simulink model "sgMdl_IO624_SyncAsync"  (R2024b)
settings: Solver=FixedStepAuto  StartTime=0.0  StopTime=inf  RelTol=1e-3  EnableMultiTasking=on
undefined symbols (not defined in the file): A, Asynchronous, FIFO, ns, PSI5, Triggered, us
libraries: speedgoatlib_IO624 x7
Description:
  | IO624 - PSI5
settings Model: ModifiedByFormat=Speedgoat  SimulationMode=external  ExtModeEnableFloating=off  ExtModeTrigDuration=100000  Creator=Speedgoat  LastModifiedBy=Speedgoat
settings SolverCC: ConcurrentTasks=on  AlgebraicLoopSolver=TrustRegion  PositivePriorityOrder=on  AutoInsertRateTranBlk=on  InsertRTBMode=Never (minimum delay)
settings DataIOCC: SaveFormat=StructureWithTime
settings OptimizationCC: BlockReduction=off  OptimizeBlockIOStorage=off  BufferReuse=off  GlobalBufferReuse=off  ExpressionFolding=off  LocalBlockOutputs=off  OptimizeDataStoreBuffers=off  BusAssignmentInplaceUpdate=off
settings DebuggingCC: InheritedTsInSrcMsg=none  TasksWithSamePriorityMsg=none  ParameterPrecisionLossMsg=none  UnconnectedInputMsg=warning  UnconnectedOutputMsg=warning  UnconnectedLineMsg=warning
settings HardwareCC: ProdBitPerLong=64  ProdLongLongMode=on  ProdHWDeviceType=Intel->x86-64 (Linux 64)
settings ModelReferenceCC: EnableRefExpFcnMdlSchedulingChecks=on
settings SFSimCC: CustomCodeUndefinedFunction=UseInterfaceOnly
settings RTWCC: Description=Speedgoat Real-Time Target Machine  SystemTargetFile=speedgoat.tlc  TemplateMakefile=slrealtime_default_tmf  PostCodeGenCommand=sg.model.build.makeCfg(bdroot, buildInfo);  Toolchain=Simulink Real-Time Toolchain  BuildConfiguration=Faster Runs  TargetLang=C++  GPUComputeCapability=3.5  DLArmComputeVersion=19.05
settings SimulinkRealTimeTargetCC: SubcomponentCodeInterfacePackaging=Reusable function  InstructionSetFMA=off  LogToMDFFile=off  SLRTFileLogMaxRuns=10
settings ConfigComp: CovBoundaryAbsTol=1.0e-5

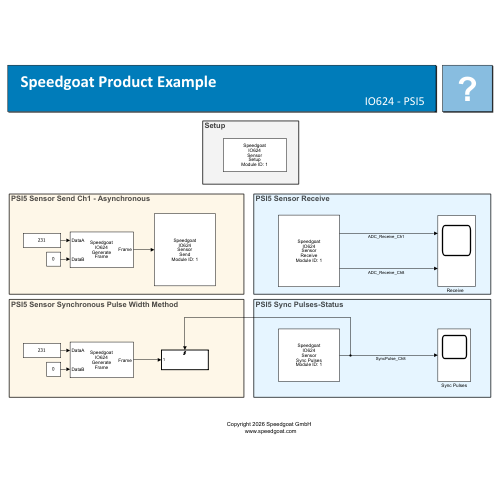
[thumbnail: Simulink's stored preview of the top-level diagram]
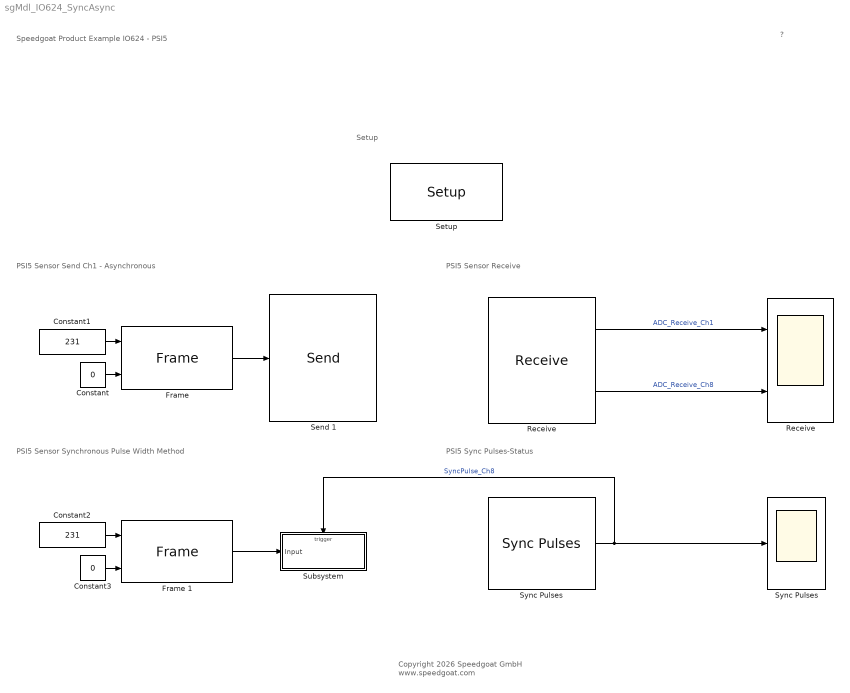
== system sgMdl_IO624_SyncAsync ==
  note: Setup
  note: PSI5 Sensor Send Ch1 - Asynchronous
  note: PSI5 Sensor Receive
  note: PSI5 Sensor Synchronous Pulse Width Method
  note: PSI5 Sync Pulses-Status
  note: Speedgoat Product Example
      | IO624 - PSI5
  note: ?
  note: Copyright 2026 Speedgoat GmbH
      |  www.speedgoat.com
  Constant : Constant  Value=0  OutDataTypeStr=uint16
  Constant1 : Constant  Value=231  OutDataTypeStr=uint32
  Constant2 : Constant  Value=231  OutDataTypeStr=uint32
  Constant3 : Constant  Value=0  OutDataTypeStr=uint16
  "Frame " : speedgoatlib_IO624/Frame   parSizeDataA=7  parSizeDataB=0  parEnableMsging=off  parMsging=[1, 1]  parEnableFrameCtrl=off  parFrameCtrl=[1, 0]  parEnableMsgStatus=off  parMsgStatus=[0, 1]
      settings: SourceProductName=IO624
  Frame 1 : speedgoatlib_IO624/Frame   parSizeDataA=7  parSizeDataB=0  parEnableMsging=off  parMsging=[1, 1]  parEnableFrameCtrl=off  parFrameCtrl=[1, 0]  parEnableMsgStatus=off  parMsgStatus=[0, 1]
      settings: SourceProductName=IO624
  "Receive " : speedgoatlib_IO624/Receive   parModuleId=1  parModuleNumber=624  parSampleTime=5e-5  parPciSlot=-1  parMonitorCh=[1 8]
      settings: SourceProductName=IO624
  "Receive  " : Scope  NumInputPorts=2
  Send 1 : speedgoatlib_IO624/Send   parSendChannels=1  parModuleNumber=624  parModuleId=1  parSampleTime=5e-5  parSendChStatus1=off  parSendChStatus2=off  parSendChStatus3=off  parSendChStatus4=off  parSendChStatus5=off  parSendChStatus6=off  parSendChStatus7=off  parSendChStatus8=off  parSendChannel1=on  parSendChannel2=off  parSendChannel3=off  parSendChannel4=off  parSendChannel5=off  parSendChannel6=off  parSendChannel7=off  parSendChannel8=off  parPciSlot=-1  parCtrChannels=[2 1 1 1 1 1 1 2]  parSendChsStatus=zeros(1,0)  parSendPSI5=[1 1 1 1 2 2 2 2 105 105 105 105 65 65 65 65 1000 500 500 500 500 500 500 1500]
      settings: SourceProductName=IO624
  "Setup " : speedgoatlib_IO624/Setup   parModuleNumber=624  parModuleId=1  parPciSlot=-1  parTriggerSignal=TTL  parChsequence=[1 8]  parCtrChannels=[2 1 1 1 1 1 1 2]  parCtrCh1=PSI5 Sensor Emulator  parMonitorCh1=on  parCtrCh2=Disabled  parMonitorCh2=off  parCtrCh3=Disabled  parMonitorCh3=off  parCtrCh4=Disabled  parMonitorCh4=off  parCtrCh5=Disabled  parMonitorCh5=off  parCtrCh6=Disabled  parMonitorCh6=off  parCtrCh7=Disabled  parMonitorCh7=off  parCtrCh8=PSI5 Sensor Emulator  parMonitorCh8=on  parModuleSetV=[1 2 1 1 1 1 1 1 2]  parCurrentL=[0 14000 10000 0 14000 10000 0 14000 10000 0 14000 10000 10000 14000 17000 10000 14000 17000 10000 14000 17000 10000 14000 17000 0 0 0]  parCh1=[0 0 80 0 0 1000 8600 3000 5 45 2 0 0 0 1 10 1 1]  parCh2=[0 0 0 0 0 0 0 0 0 0 0 0 0 0 0 0 0 0]  parCh3=[0 0 0 0 0 0 0 0 0 0 0 0 0 0 0 0 0 0]  parCh4=[0 0 0 0 0 0 0 0 0 0 0 0 0 0 0 0 0 0]  parCh5=[0 0 0 0 0 0 0 0 0 0 0 0 0 0 0 0 0 0]  parCh6=[0 0 0 0 0 0 0 0 0 0 0 0 0 0 0 0 0 0]  parCh7=[0 0 0 0 0 0 0 0 0 0 0 0 0 0 0 0 0 0]  parCh8=[0 0 80 0 0 1500 8600 3000 5 645 2 0 0 0 1 5 2 1]  parPSI5BusModeCh1=PSI5-A (Asynchronous)  parPSI5NBitsCh1=10  parPSI5SBEnableCh1=Start Bit Enable  parPSI5StartBitSXCh1=[0, 0]  parPSI5DataDTCh1=105  parPSI5PayloadCrcCh1=1  parPSI5UVRCh1=Disable  parPSI5UnderVoltReVTHCh1=3000  psi5ReDetecTimeTTHCh1=5  parPSI5SlotDCh1=45  parPSI5PulseModeCh1=Pulse Width Method  parPSI5FrameLCh1=Frame 2a Long (Nibble)  parPSI5SSVoltageCh1=8600  parAKASpeedPulseCh1=Normal (High Current)  parEnDynSpeedPulseLvlCh1=on  parCustomModeCh1=FIFO-Triggered  parCustomNrFifoFramesCh1=1  parBitRateCh1=125 kbps  parBitTimeBaseCh1=0.1 [us]  parBitTimeFactorCh1=80  textEffBitTimeCh1=8.0 [us]  parPulseTimeBaseCh1="50  [ns]"  parPulseTimeFactorCh1=8  textEffPulseTimeCh1=400.0 [ns]  parCycleTimeDesiredCh1=Choose with Time Base and Time Factor  parCycleTimeBaseCh1="1    [us]"  parCycleTimeFactorCh1=1000  textEffCycleTimeCh1=1000.0 [us]  parEnDynTimingCh1=off  parCLCSettingCh1=Custom  parCLHighCh1=10000  parCLMidCh1=14000  parCLLowCh1=0  parPSI5BusModeCh2=PSI5-A (Asynchronous)  parPSI5NBitsCh2=10  parPSI5SBEnableCh2=Start Bit Enable  parPSI5StartBitSXCh2=[0, 0]  parPSI5DataDTCh2=105  parPSI5PayloadCrcCh2=1  parPSI5UVRCh2=Disable  parPSI5UnderVoltReVTHCh2=3000  psi5ReDetecTimeTTHCh2=5  parPSI5SlotDCh2=0  parPSI5PulseModeCh2=Tooth Gap Method  parPSI5FrameLCh2=Frame 2a Long (Nibble)  parPSI5SSVoltageCh2=0  parAKASpeedPulseCh2=Normal (High Current)  parEnDynSpeedPulseLvlCh2=off  parCustomModeCh2=FIFO-Triggered  parCustomNrFifoFramesCh2=1  parBitRateCh2=125 kbps  parBitTimeBaseCh2=0.1 [us]  parBitTimeFactorCh2=80  textEffBitTimeCh2=8.0 [us]  parPulseTimeBaseCh2="50  [ns]"  parPulseTimeFactorCh2=8  textEffPulseTimeCh2=400.0 [ns]  parCycleTimeDesiredCh2=Choose with Time Base and Time Factor  parCycleTimeBaseCh2="50  [ns]"  parCycleTimeFactorCh2=500  textEffCycleTimeCh2=25000.0 [ns]  parEnDynTimingCh2=off  parCLCSettingCh2=Custom  parCLHighCh2=10000  parCLMidCh2=14000  parCLLowCh2=0  parPSI5BusModeCh3=PSI5-A (Asynchronous)  parPSI5NBitsCh3=10  parPSI5SBEnableCh3=Start Bit Enable  parPSI5StartBitSXCh3=[0, 0]  parPSI5DataDTCh3=105  parPSI5PayloadCrcCh3=487  parPSI5UVRCh3=Disable  parPSI5UnderVoltReVTHCh3=3000  psi5ReDetecTimeTTHCh3=5  parPSI5SlotDCh3=0  parPSI5PulseModeCh3=Tooth Gap Method  parPSI5FrameLCh3=Frame 2a Long (Nibble)  parPSI5SSVoltageCh3=0  parAKASpeedPulseCh3=Normal (High Current)  parEnDynSpeedPulseLvlCh3=off  parCustomModeCh3=FIFO-Triggered  parCustomNrFifoFramesCh3=1  parBitRateCh3=125 kbps  parBitTimeBaseCh3=0.1 [us]  parBitTimeFactorCh3=80  textEffBitTimeCh3=8.0 [us]  parPulseTimeBaseCh3=0.1 [us]  parPulseTimeFactorCh3=8  textEffPulseTimeCh3=0.8 [us]  parCycleTimeDesiredCh3=Choose with Time Base and Time Factor  parCycleTimeBaseCh3="50  [ns]"  parCycleTimeFactorCh3=500  textEffCycleTimeCh3=25000.0 [ns]  parEnDynTimingCh3=off  parCLCSettingCh3=Custom  parCLHighCh3=10000  parCLMidCh3=14000  parCLLowCh3=0  parPSI5BusModeCh4=PSI5-A (Asynchronous)  parPSI5NBitsCh4=10  parPSI5SBEnableCh4=Start Bit Enable  parPSI5StartBitSXCh4=[0, 0]  parPSI5DataDTCh4=105  parPSI5PayloadCrcCh4=487  parPSI5UVRCh4=Disable  parPSI5UnderVoltReVTHCh4=3000  psi5ReDetecTimeTTHCh4=5  parPSI5SlotDCh4=0  parPSI5PulseModeCh4=Tooth Gap Method  parPSI5FrameLCh4=Frame 2a Long (Nibble)  parPSI5SSVoltageCh4=0  parAKASpeedPulseCh4=Normal (High Current)  parEnDynSpeedPulseLvlCh4=off  parCustomModeCh4=FIFO-Triggered  parCustomNrFifoFramesCh4=1  parBitRateCh4=Custom  parBitTimeBaseCh4=0.1 [us]  parBitTimeFactorCh4=80  textEffBitTimeCh4=8.0 [us]  parPulseTimeBaseCh4="50  [ns]"  parPulseTimeFactorCh4=8  textEffPulseTimeCh4=400.0 [ns]  parCycleTimeDesiredCh4=Choose with Time Base and Time Factor  parCycleTimeBaseCh4="50  [ns]"  parCycleTimeFactorCh4=500  textEffCycleTimeCh4=25000.0 [ns]  parEnDynTimingCh4=off  parCLCSettingCh4=Custom  parCLHighCh4=10000  parCLMidCh4=14000  parCLLowCh4=0  parPSI5BusModeCh5=PSI5-U/P (Synchronous without Daisy Chain)  parPSI5NBitsCh5=5  parPSI5SBEnableCh5=Start Bit Enable  parPSI5StartBitSXCh5=[0, 0]  parPSI5DataDTCh5=65  parPSI5PayloadCrcCh5=487  parPSI5UVRCh5=Disable  parPSI5UnderVoltReVTHCh5=3000  psi5ReDetecTimeTTHCh5=5  parPSI5SlotDCh5=0  parPSI5PulseModeCh5=Pulse Width Method  parPSI5FrameLCh5=Frame 2a Long (Nibble)  parPSI5SSVoltageCh5=8600  parAKASpeedPulseCh5=Normal (High Current)  parEnDynSpeedPulseLvlCh5=off  parCustomModeCh5=FIFO-Triggered  parCustomNrFifoFramesCh5=1  parBitRateCh5=125 kbps  parBitTimeBaseCh5=0.1 [us]  parBitTimeFactorCh5=80  textEffBitTimeCh5=8.0 [us]  parPulseTimeBaseCh5="50  [ns]"  parPulseTimeFactorCh5=8  textEffPulseTimeCh5=400.0 [ns]  parCycleTimeDesiredCh5=Choose with Time Base and Time Factor  parCycleTimeBaseCh5="50  [ns]"  parCycleTimeFactorCh5=500  textEffCycleTimeCh5=25000.0 [ns]  parEnDynTimingCh5=off  parCLCSettingCh5=Custom  parCLHighCh5=17000  parCLMidCh5=14000  parCLLowCh5=10000  parPSI5BusModeCh6=PSI5-U/P (Synchronous without Daisy Chain)  parPSI5NBitsCh6=5  parPSI5SBEnableCh6=Start Bit Enable  parPSI5StartBitSXCh6=[0, 0]  parPSI5DataDTCh6=65  parPSI5PayloadCrcCh6=487  parPSI5UVRCh6=Disable  parPSI5UnderVoltReVTHCh6=3000  psi5ReDetecTimeTTHCh6=5  parPSI5SlotDCh6=645  parPSI5PulseModeCh6=Pulse Width Method  parPSI5FrameLCh6=Frame 2a Long (Nibble)  parPSI5SSVoltageCh6=8600  parAKASpeedPulseCh6=Normal (High Current)  parEnDynSpeedPulseLvlCh6=off  parCustomModeCh6=FIFO-Triggered  parCustomNrFifoFramesCh6=1  parBitRateCh6=125 kbps  parBitTimeBaseCh6=0.1 [us]  parBitTimeFactorCh6=80  textEffBitTimeCh6=8.0 [us]  parPulseTimeBaseCh6="50  [ns]"  parPulseTimeFactorCh6=8  textEffPulseTimeCh6=400.0 [ns]  parCycleTimeDesiredCh6=Choose with Time Base and Time Factor  parCycleTimeBaseCh6="50  [ns]"  parCycleTimeFactorCh6=500  textEffCycleTimeCh6=25000.0 [ns]  parEnDynTimingCh6=off  parCLCSettingCh6=Custom  parCLHighCh6=17000  parCLMidCh6=14000  parCLLowCh6=10000  parPSI5BusModeCh7=PSI5-U/P (Synchronous without Daisy Chain)  parPSI5NBitsCh7=5  parPSI5SBEnableCh7=Start Bit Enable  parPSI5StartBitSXCh7=[0, 0]  parPSI5DataDTCh7=65  parPSI5PayloadCrcCh7=1  parPSI5UVRCh7=Disable  parPSI5UnderVoltReVTHCh7=3000  psi5ReDetecTimeTTHCh7=5  parPSI5SlotDCh7=0  parPSI5PulseModeCh7=Pulse Width Method  parPSI5FrameLCh7=Frame 2a Long (Nibble)  parPSI5SSVoltageCh7=8600  parAKASpeedPulseCh7=Normal (High Current)  parEnDynSpeedPulseLvlCh7=off  parCustomModeCh7=FIFO-Triggered  parCustomNrFifoFramesCh7=1  parBitRateCh7=125 kbps  parBitTimeBaseCh7=0.1 [us]  parBitTimeFactorCh7=80  textEffBitTimeCh7=8.0 [us]  parPulseTimeBaseCh7="50  [ns]"  parPulseTimeFactorCh7=8  textEffPulseTimeCh7=400.0 [ns]  parCycleTimeDesiredCh7=Choose with Time Base and Time Factor  parCycleTimeBaseCh7="50  [ns]"  parCycleTimeFactorCh7=500  textEffCycleTimeCh7=25000.0 [ns]  parEnDynTimingCh7=off  parCLCSettingCh7=Custom  parCLHighCh7=17000  parCLMidCh7=14000  parCLLowCh7=10000  parPSI5BusModeCh8=PSI5-U/P (Synchronous without Daisy Chain)  parPSI5NBitsCh8=5  parPSI5SBEnableCh8=Start Bit Enable  parPSI5StartBitSXCh8=[0, 0]  parPSI5DataDTCh8=65  parPSI5PayloadCrcCh8=1  parPSI5UVRCh8=Disable  parPSI5UnderVoltReVTHCh8=3000  psi5ReDetecTimeTTHCh8=5  parPSI5SlotDCh8=645  parPSI5PulseModeCh8=Pulse Width Method  parPSI5FrameLCh8=Frame 2a Long (Nibble)  parPSI5SSVoltageCh8=8600  parAKASpeedPulseCh8=Normal (High Current)  parEnDynSpeedPulseLvlCh8=off  parCustomModeCh8=FIFO-Triggered  parCustomNrFifoFramesCh8=1  parBitRateCh8=125 kbps  parBitTimeBaseCh8=0.1 [us]  parBitTimeFactorCh8=80  textEffBitTimeCh8=8.0 [us]  parPulseTimeBaseCh8="50  [ns]"  parPulseTimeFactorCh8=8  textEffPulseTimeCh8=400.0 [ns]  parCycleTimeDesiredCh8=Choose with Time Base and Time Factor  parCycleTimeBaseCh8="1    [us]"  parCycleTimeFactorCh8=1500  textEffCycleTimeCh8=1500.0 [us]  parEnDynTimingCh8=off  parCLCSettingCh8=Custom  parCLHighCh8=17000  parCLMidCh8=14000  parCLLowCh8=10000
      settings: SourceProductName=IO624
  Subsystem : Subsystem
  Sync Pulses : Scope
  "Sync Pulses " : speedgoatlib_IO624/Sync Pulses   parPciSlot=-1  parMonitorCh=[1 2]  parSyncCh=8  parPSI5PulseModeCh=[2 1 1 1 2 2 2 2]  parPSI5FrameLCh=[1 1 1 1 1 1 1 1]  parPSI5BusModeCh=[1 1 1 1 2 2 2 2]  parChData=1  parModuleId=1  parModuleNumber=624  parSampleTime=-1  parChData1=on  parChData2=off  parChData3=off  parChData4=off  parChData5=off  parChData6=off  parChData7=off  parChData8=off  parChData9=off
      settings: SourceProductName=IO624
  wires:
  "Receive "/1 -> "Receive  "/1  "ADC_Receive_Ch1"
  "Receive "/2 -> "Receive  "/2  "ADC_Receive_Ch8"
  "Sync Pulses "/1 -> Sync Pulses/1, Subsystem/Trigger  "SyncPulse_Ch8"
  "Frame "/1 -> Send 1/1
  Constant1/1 -> "Frame "/1
  Constant2/1 -> Frame 1/1
  Frame 1/1 -> Subsystem/1(Input)
  Constant/1 -> "Frame "/2
  Constant3/1 -> Frame 1/2

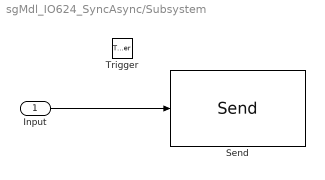
== system sgMdl_IO624_SyncAsync/Subsystem ==
  Input : Inport
  Trigger : TriggerPort  VariantControl=Variant  PortDimensions=1
  "Send " : speedgoatlib_IO624/Send   parSendChannels=8  parModuleNumber=624  parModuleId=1  parSampleTime=-1  parSendChStatus1=off  parSendChStatus2=off  parSendChStatus3=off  parSendChStatus4=off  parSendChStatus5=off  parSendChStatus6=off  parSendChStatus7=off  parSendChStatus8=off  parSendChannel1=off  parSendChannel2=off  parSendChannel3=off  parSendChannel4=off  parSendChannel5=off  parSendChannel6=off  parSendChannel7=off  parSendChannel8=on  parPciSlot=-1  parCtrChannels=[2 1 1 1 1 1 1 2]  parSendChsStatus=zeros(1,0)  parSendPSI5=[1 1 1 1 2 2 2 2 105 105 105 105 65 65 65 65 1000 500 500 500 500 500 500 1500]
      settings: SourceProductName=IO624
  wires:
  Input/1 -> "Send "/1
